simulink model "Project1_Option3"  (R2024b)
settings: Solver=ode4  StartTime=0.0  StopTime=25  FixedStep=1  RelTol=1e-3
values from neighbouring files (symbols this model uses):
  b1 = 1    [Part2_Option1_Code.m]    (also in Part2_Option3_Code.m; Part2_option2_code.m)
  b2 = 1    [Part2_Option1_Code.m]    (also in Part2_Option3_Code.m; Part2_option2_code.m)
  J1 = 100    [Part2_Option1_Code.m]    (also in Part2_Option3_Code.m; Part2_option2_code.m; Project1_Part1_Code_revision_1.m = [100, 0.01]; Project1_Part1_Code_revision_current.m = [100, 0.01])
  J2 = 1    [Part2_Option1_Code.m]    (also in Part2_Option3_Code.m; Part2_option2_code.m)
  omega_init = [10,0]    [Part2_Option1_Code.m]    (also in Part2_Option3_Code.m; Part2_option2_code.m; Project1_Part1_Code_revision_1.m; Project1_Part1_Code_revision_current.m)
  tau = [0, 100]    [Part2_option2_code.m]    (also in Project1_Part1_Code_revision_1.m; Project1_Part1_Code_revision_current.m)
  theta0 = 0    [P1.m]    (also in Part2_Option1_Code.m; Part2_Option3_Code.m; Part2_option2_code.m; Project1_Part1_Code_revision_1.m)
  w = simOut.omega.Data    [P1.m]
undefined symbols (not defined in the file or in its folder): torque
settings Model: Creator=jacobcody  LastModifiedBy=jacobcody

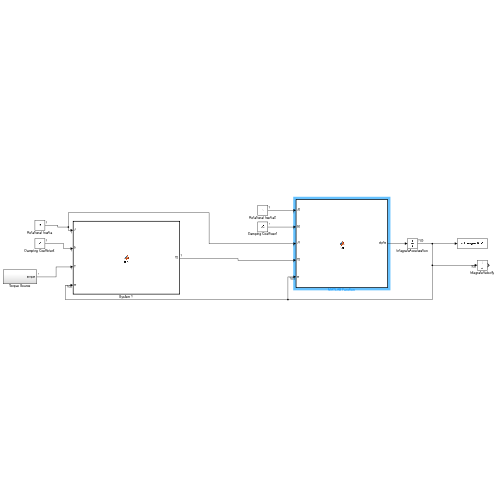
[thumbnail: Simulink's stored preview of the top-level diagram]
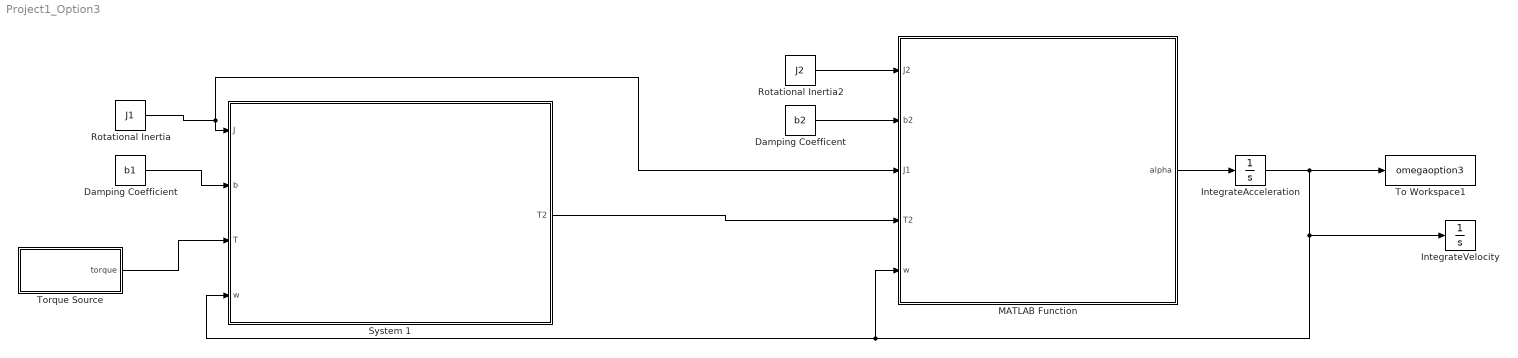
== system Project1_Option3 ==
  Damping Coefficent : Constant  Value=b2
  Damping Coefficient : Constant  Value=b1
  IntegrateAcceleration : Integrator  InitialCondition=omega_init
  IntegrateVelocity : Integrator  InitialCondition=theta0
  MATLAB Function : MATLAB Function  TreatAsAtomicUnit=on
  Rotational Inertia : Constant  Value=J1
  Rotational Inertia2 : Constant  Value=J2
  System 1 : MATLAB Function  TreatAsAtomicUnit=on
  To Workspace1 : ToWorkspace  VariableName=omegaoption3  SaveFormat=Timeseries  SampleTime=-1
  Torque Source : Subsystem
  wires:
  Rotational Inertia/1 -> MATLAB Function/3(J1), System 1/1(J)
  Damping Coefficient/1 -> System 1/2(b)
  System 1/1(T2) -> MATLAB Function/4(T2)
  Rotational Inertia2/1 -> MATLAB Function/1(J2)
  Damping Coefficent/1 -> MATLAB Function/2(b2)
  MATLAB Function/1(alpha) -> IntegrateAcceleration/1
  IntegrateAcceleration/1 -> MATLAB Function/5(w), System 1/4(w), IntegrateVelocity/1, To Workspace1/1
  Torque Source/1(torque) -> System 1/3(T)

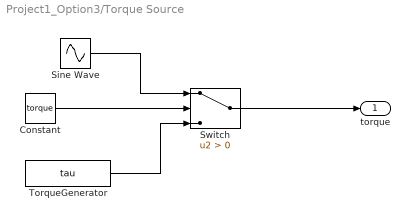
== system Project1_Option3/Torque Source ==
  Constant : Constant  Value=torque
  Sine Wave : Sin  Frequency=w  SampleTime=0
  Switch : Switch  Criteria=u2 > Threshold  SaturateOnIntegerOverflow=off  InputSameDT=off
  TorqueGenerator : Constant  Value=tau
  torque : Outport
  wires:
  Switch/1 -> torque/1
  Sine Wave/1 -> Switch/1
  TorqueGenerator/1 -> Switch/3
  Constant/1 -> Switch/2

== matlab function Project1_Option3/MATLAB Function ==
  data: J2 input; alpha output; b2 input; J1 input; T2 input; w input
function alpha = fcn(J2,b2,J1,T2,w)
alpha =(1/(J1+J2)*(T2-T1)-(((b2)/(J1+J2))*w));

== matlab function Project1_Option3/System 1 ==
  data: J input; b input; T input; w input; T2 output
function  T2= fcn(J,b,T,w)
T2=T ;%-(w*b)-(J*wdot)
